simulink library "bcm"  (R2021b)
settings: Solver=VariableStepAuto  StartTime=0.0  StopTime=10.0  RelTol=1e-3
undefined symbols (not defined in the file or in its folder): ENUM_ANTITHEFT_ALARM, ENUM_ANTITHEFT_ARM, ENUM_ANTITHEFT_DISARM, ENUM_ANTITHEFT_WAIT, ENUM_GEARPOSNTOCAN_P, ENUM_PDKEYRAWLULOCK_INUNLOCK, ENUM_PDKEYRAWPS_INPS, ENUM_POWERSTA_ON, ENUM_POWERSTA_READY, ENUM_POWERSTA_STANDBY, ENUM_PWRSTASW_ON, ENUM_PWRSTASW_READY, ENUM_VEHICLETYPE_D21, ENUM_VEHICLETYPE_D31F25, ENUM_VEHICLETYPE_D31HAWD, ENUM_VEHICLETYPE_D31HRWD, ENUM_VEHICLETYPE_D31L24, FALSE, KBCM_ACCSwcPrsTmr_s, KBCM_ALMBrightnessDark_enum, KBCM_AmbBlue_enum, KBCM_AmbBreathT_ms, KBCM_AmbGreen_enum, KBCM_AmbMidPple_enum, KBCM_AmbRed_enum, KBCM_AmbTempCtrlEN_flg, KBCM_AmbTempT_s, KBCM_AmbWelModeENWait_s, KBCM_Antitheft_enum_ovrdflg, KBCM_Antitheft_enum_ovrdval, KBCM_APMDoorCtrlSta_flg_ovrdflg, KBCM_APMDoorCtrlSta_flg_ovrdval, KBCM_CmdKeepT_s, KBCM_CSWLightRstDebT_s, KBCM_CSWTurnLPRstT_s, KBCM_DelayTSW_flg, KBCM_DiagDRLOFF_flg, KBCM_DiagFLTC_mA, KBCM_DiagFMHT_s, KBCM_DiagFRTC_mA, KBCM_DiagRLTC_mA, KBCM_DiagRRTC_mA, KBCM_DrAPMRetryTimes_cnt, KBCM_DrOpenWdwOT_s, KBCM_DrOpenWdwReady_s, KBCM_ESSOffT_ms, KBCM_ESSOnT_ms, KBCM_FDCDKCReDetectT_K, KBCM_FDCDKCUSSFilterT_K, KBCM_HandleLampKeepT_s, KBCM_IVIRstHoldT_ms, KBCM_IVIRstTriggerT_ms, KBCM_ONDelayT_ms, KBCM_RAPSAbnFlashOFFT_ms, KBCM_RAPSAbnFlashONT_ms, KBCM_ReDetectT_K, KBCM_RightHandDriveEN_flg, KBCM_RLSLowSpdFilterT_s, KBCM_RmLampKeep_min, KBCM_RmLpKeyInT_s ... (+37)
libraries: simulink x389, $bdroot x11, hcu_lib x2
(part 13 of 13)

== stateflow chart bcm/BCM/BCM/Amb/AmbientLight ==
  state TempControl [parallel]
    settings: executionOrder=12
    state TempUP
      en:VBCM_AmbTemp_enum=1;
    state Wait
    state StandBy
      en:VBCM_AmbTemp_enum=0;
    state TempDN
      en:VBCM_AmbTemp_enum=2;
    (default) -> TempControl.StandBy
    TempControl -> TempUP [order 1] : [hasChanged(VBCM_TempUP_flg) && VBCM_TempUP_flg]
    TempUP -> TempControl.Wait : [!VBCM_TempUP_flg]
    TempControl.Wait -> TempControl.StandBy : [after(KBCM_AmbTempT_s,tick)]
    TempDN -> TempControl.Wait : [!VBCM_TempDN_flg]
    TempControl -> TempDN [order 2] : [hasChanged(VBCM_TempDN_flg) && VBCM_TempDN_flg]
  state OutputColor [parallel]
    settings: executionOrder=1
    (default) -> (junction 25)
    OutputColor -> (junction 25)
    (junction 25) -> (junction 947) [order 1] : [VINP_AmbLinkDriSta_flg]
    (junction 947) -> (junction 948) [order 1] : [VINP_IVISnowModeCmd_flg == 1]
        | {VBCM_AmbLightColor_enum = KBCM_AmbMidPurple_enum;}
    (junction 25) -> (junction 200) [order 2] : {VBCM_AmbLightColor_enum=VINP_AmbColorSta_enum;}
    (junction 947) -> (junction 28) [order 2]
    (junction 28) -> (junction 33) [order 1] : [VINP_IVIPWModeReq_enum==1]....
        | {VBCM_AmbLightColor_enum=KBCM_AmbRed_enum;}
    (junction 28) -> (junction 35) [order 2]
    (junction 35) -> (junction 37) [order 1] : [VINP_IVIPWModeReq_enum==2]....
        | {VBCM_AmbLightColor_enum=KBCM_AmbGreen_enum;}
    (junction 35) -> (junction 39) [order 2]
    (junction 39) -> (junction 41) : {VBCM_AmbLightColor_enum=KBCM_AmbBlue_enum;}
  state LampPower [parallel]
    settings: executionOrder=4
    state LampON
      state WaitForLampPwrON
        en:VBCM_LampPwr_flg=1;
      state LampPwrON
        en:VBCM_LampPwrReady_flg=true;
      (default) -> WaitForLampPwrON
      WaitForLampPwrON -> LampPwrON : after(5,tick)
    state OFF
      en:VBCM_LampPwr_flg=0;
      VBCM_LampPwrReady_flg=false;
    (default) -> LampPower.OFF
    LampPower.OFF -> LampON : [VBCM_WakeUp_flg==1||VPMM_PwrSta_enum>0]
    LampON -> LampPower.OFF : [VBCM_WakeUp_flg==0&&VPMM_PwrSta_enum==0]
  state WelcomeModeEnable [parallel]
    settings: executionOrder=13
    state WelcomeModeDisable
      en:
      VBCM_WelcomrModeEN_flg = FALSE;
    state WelcomrModeEnable
      state Wait
      state Enable
        en:
        VBCM_WelcomrModeEN_flg = TRUE;
      (default) -> WelcomeModeEnable.WelcomrModeEnable.Wait
      WelcomeModeEnable.WelcomrModeEnable.Wait -> Enable : [after(KBCM_AmbWelModeENWait_s, tick)]
    (default) -> WelcomeModeDisable
    WelcomeModeDisable -> WelcomeModeEnable.WelcomrModeEnable.Wait : [VPMM_PwrSta_enum > 3]
    WelcomrModeEnable -> WelcomeModeDisable : [VPMM_PwrSta_enum <= 3]
  state SOCDet [parallel]
    settings: executionOrder=5
    state ON
      state SOCOK
        en:SOCWarning=0;
      state SOCWarning1
      state SOCWarning2
        en:SOCWarning=1;
      (default) -> (junction 516)
      (junction 516) -> SOCOK [order 1] : [VINP_HVBattSOCDis_pct>5]
      (junction 516) -> (junction 518) [order 2]
      SOCOK -> SOCWarning1 : [VINP_HVBattSOCDis_pct<=5]....
          | {SOCWarning=1;}
      SOCWarning1 -> SOCOK [order 1] : [VINP_HVBattSOCDis_pct>5]
      (junction 518) -> SOCWarning1 [order 1] : [VINP_HVBattSOCDis_pct>=1]....
          | {SOCWarning=1;}
      (junction 518) -> (junction 521) [order 2]
      SOCWarning2 -> SOCWarning1 : [VINP_HVBattSOCDis_pct>=1]
      SOCWarning1 -> SOCWarning2 [order 2] : [VINP_HVBattSOCDis_pct<1]
      (junction 521) -> SOCWarning2
    state OFF
      en:SOCWarning=0;
    (default) -> SOCDet.OFF
    SOCDet.OFF -> SOCDet.ON : [VINP_AmbFunEN_flg&&....
        | VINP_AmbPwrWarnEN_flg]
    SOCDet.ON -> SOCDet.OFF : [!VINP_AmbPwrWarnEN_flg||....
        | !VINP_AmbFunEN_flg]
  state OutputBrightness [parallel]
    settings: executionOrder=3
    state ON
      (default) -> (junction 92)
      OutputBrightness.ON -> (junction 92) [order 1] : [VBCM_LampPwrReady_flg]
      (junction 92) -> (junction 90) [order 1] : [VINP_IVINightModeSta_flg&&VBCM_PosLamp_flg||VPMM_PwrSta_enum<=3]....
          | {VBCM_AmbLightBrightness_enum=KBCM_ALMBrightnessDark_enum;}
      (junction 92) -> (junction 203) [order 2]
      (junction 203) -> (junction 324) [order 1] : [!VINP_IVINightModeSta_flg&&VBCM_PosLamp_flg&&VINP_AmbDimEN_flg]....
          | {VBCM_AmbLightBrightness_enum=VINP_AmbBrightnessSta_enum/2;}
      (junction 203) -> (junction 208) [order 2] : {VBCM_AmbLightBrightness_enum=VINP_AmbBrightnessSta_enum;}
    state OFF
      en:VBCM_AmbLightBrightness_enum=0;
    (default) -> OutputBrightness.OFF
    OutputBrightness.OFF -> OutputBrightness.ON : [VINP_AmbFunEN_flg]
    OutputBrightness.ON -> OutputBrightness.OFF [order 1] : [!VINP_AmbFunEN_flg]
  state WelcomeMode [parallel]
    settings: executionOrder=2
    state Arm
      en:VBCM_Welcome_flg=0;
    state Disarm
      state WaitForDoorOpen
      state WaitForWelcomeModeEN
      state DoorOpen
        en:
        VBCM_Welcome_flg=1;
        on after(KBCM_AmbBreathT_tick,tick):
        VBCM_Welcome_flg=0;
      (default) -> (junction 498)
      (junction 498) -> WaitForDoorOpen [order 2]
      (junction 498) -> WaitForWelcomeModeEN [order 1] : [VINP_AllDoorSW_flg || ....
          | VPMM_PwrSta_enum>3]
      WaitForDoorOpen -> WaitForWelcomeModeEN : [VINP_AllDoorSW_flg || ....
          | VPMM_PwrSta_enum>3]
      WaitForWelcomeModeEN -> DoorOpen : [VBCM_WelcomrModeEN_flg]
    (default) -> (junction 492)
    (junction 492) -> Disarm [order 1] : [EEP_AntitheftSta==0]
    (junction 492) -> Arm [order 2]
    Arm -> Disarm : [AntitheftSta==0]
    Disarm -> Arm : [AntitheftSta!=0]
  state WarningLamp1 [parallel]
    settings: executionOrder=11
    state StandBy
    state Wait
    (default) -> (junction 549)
    WarningLamp1.StandBy -> (junction 549)
    (junction 549) -> (junction 504)
    (junction 545) -> WarningLamp1.StandBy
    (junction 504) -> (junction 545) [order 1] : [VINP_AmbFunEN_flg&&VBCM_Welcome_flg&&VINP_AmbWelEN_flg]{VBCM_AmblightBreath1_enum=1;}
    (junction 504) -> (junction 527) [order 2]
    (junction 543) -> (junction 545)
    WarningLamp1.Wait -> (junction 543) : [after(KBCM_AmbBreathT_tick,tick)]
    (junction 527) -> WarningLamp1.Wait [order 1] : [VINP_AmbFunEN_flg&&SOCWarning==1]....
        | {SOCWarning=0;VBCM_AmblightBreath1_enum=2;}
    (junction 527) -> (junction 900) [order 2]
    (junction 903) -> (junction 543)
    (junction 900) -> (junction 903) [order 1] : [VINP_VehicleType_enum != ENUM_VEHICLETYPE_D31L24 && ...
        | VINP_AmbFunEN_flg && KBCM_AmbTempCtrlEN_flg && VBCM_AmbTemp_enum==1]
        | {VBCM_AmblightBreath1_enum =4 ;}
    (junction 900) -> (junction 901) [order 2]
    (junction 902) -> (junction 903)
    (junction 901) -> (junction 902) [order 1] : [VINP_VehicleType_enum != ENUM_VEHICLETYPE_D31L24 && ...
        | VINP_AmbFunEN_flg && KBCM_AmbTempCtrlEN_flg && VBCM_AmbTemp_enum==2]
        | {VBCM_AmblightBreath1_enum =5 ;}
    (junction 901) -> (junction 537) [order 2]
    (junction 542) -> (junction 902)
    (junction 537) -> (junction 542) : {SOCWarning=0;VBCM_AmblightBreath1_enum=0;}
  state WarningLamp3 [parallel]
    settings: executionOrder=7
    state StandBy
    state Wait
    (default) -> (junction 576)
    WarningLamp3.StandBy -> (junction 576)
    (junction 576) -> (junction 577)
    (junction 578) -> WarningLamp3.StandBy
    (junction 577) -> (junction 578) [order 1] : [VINP_AmbFunEN_flg&&VBCM_Welcome_flg&&VINP_AmbWelEN_flg]{VBCM_AmblightBreath3_enum=1;}
    (junction 577) -> (junction 597) [order 2]
    (junction 598) -> (junction 578)
    (junction 597) -> (junction 598) [order 1] : [VINP_AmbFunEN_flg&&VINP_AmbODAEN_flg&&....
        | ((VINP_SRRODASoundL_flg==1&&VBCM_FLDoorSW_flg==1)||VINP_SRRBSDWarnL_enum==2)]
        | {VBCM_AmblightBreath3_enum=3;}
    (junction 597) -> (junction 579) [order 2]
    (junction 580) -> (junction 598)
    (junction 579) -> WarningLamp3.Wait [order 1] : [VINP_AmbFunEN_flg&&SOCWarning==1]....
        | {VBCM_AmblightBreath3_enum=2;}
    WarningLamp3.Wait -> (junction 580) : [after(KBCM_AmbBreathT_tick,tick)]
    (junction 579) -> (junction 581) [order 2]
    (junction 582) -> (junction 580)
    (junction 581) -> (junction 582) : {VBCM_AmblightBreath3_enum=0;}
  state WarningLamp5 [parallel]
    settings: executionOrder=9
    state StandBy
    state Wait
    (default) -> (junction 630)
    WarningLamp5.StandBy -> (junction 630)
    (junction 630) -> (junction 631)
    (junction 632) -> WarningLamp5.StandBy
    (junction 631) -> (junction 632) [order 1] : [VINP_AmbFunEN_flg&&VBCM_Welcome_flg&&VINP_AmbWelEN_flg]{VBCM_AmblightBreath5_enum=1;}
    (junction 631) -> (junction 633) [order 2]
    (junction 634) -> (junction 632)
    (junction 633) -> (junction 634) [order 1] : [VINP_AmbFunEN_flg&&VINP_AmbODAEN_flg&&VINP_SRRODASoundL_flg==1&&VINP_RLDoorSW_flg==1]....
        | {VBCM_AmblightBreath5_enum=3;}
    (junction 633) -> (junction 635) [order 2]
    (junction 636) -> (junction 634)
    (junction 635) -> WarningLamp5.Wait [order 1] : [VINP_AmbFunEN_flg&&SOCWarning==1]....
        | {VBCM_AmblightBreath5_enum=2;}
    WarningLamp5.Wait -> (junction 636) : [after(KBCM_AmbBreathT_tick,tick)]
    (junction 635) -> (junction 637) [order 2]
    (junction 638) -> (junction 636)
    (junction 637) -> (junction 638) : {VBCM_AmblightBreath5_enum=0;}
  state WarningLamp2 [parallel]
    settings: executionOrder=6
    state StandBy
    state Wait
    (default) -> (junction 554)
    WarningLamp2.StandBy -> (junction 554)
    (junction 554) -> (junction 555)
    (junction 556) -> WarningLamp2.StandBy
    (junction 555) -> (junction 556) [order 1] : [VINP_AmbFunEN_flg&&VBCM_Welcome_flg&&VINP_AmbWelEN_flg]{VBCM_AmblightBreath2_enum=1;}
    (junction 555) -> (junction 557) [order 2]
    (junction 558) -> (junction 556)
    (junction 557) -> WarningLamp2.Wait [order 1] : [VINP_AmbFunEN_flg&&SOCWarning==1]....
        | {VBCM_AmblightBreath2_enum=2;}
    WarningLamp2.Wait -> (junction 558) : [after(KBCM_AmbBreathT_tick,tick)]
    (junction 557) -> (junction 910) [order 2]
    (junction 912) -> (junction 558)
    (junction 910) -> (junction 912) [order 1] : [VINP_VehicleType_enum != ENUM_VEHICLETYPE_D31L24 && ...
        | VINP_AmbFunEN_flg && KBCM_AmbTempCtrlEN_flg && VBCM_AmbTemp_enum==1]
        | {VBCM_AmblightBreath2_enum =4 ;}
    (junction 910) -> (junction 911) [order 2]
    (junction 913) -> (junction 912)
    (junction 911) -> (junction 913) [order 1] : [VINP_VehicleType_enum != ENUM_VEHICLETYPE_D31L24 && ...
        | VINP_AmbFunEN_flg && KBCM_AmbTempCtrlEN_flg && VBCM_AmbTemp_enum==2]
        | {VBCM_AmblightBreath2_enum =5 ;}
    (junction 911) -> (junction 559) [order 2]
    (junction 560) -> (junction 913)
    (junction 559) -> (junction 560) : {VBCM_AmblightBreath2_enum=0;}
  state WarningLamp4 [parallel]
    settings: executionOrder=8
    state StandBy
    state Wait
    (default) -> (junction 603)
    WarningLamp4.StandBy -> (junction 603)
    (junction 603) -> (junction 604)
    (junction 605) -> WarningLamp4.StandBy
    (junction 604) -> (junction 605) [order 1] : [VINP_AmbFunEN_flg&&VBCM_Welcome_flg&&VINP_AmbWelEN_flg]{VBCM_AmblightBreath4_enum=1;}
    (junction 604) -> (junction 606) [order 2]
    (junction 607) -> (junction 605)
    (junction 606) -> (junction 607) [order 1] : [VINP_AmbFunEN_flg&&VINP_AmbODAEN_flg&&....
        | ((VINP_SRRODASoundR_flg==1&&VBCM_FRDoorSW_flg==1)||VINP_SRRBSDWarnR_enum==2)]
        | {VBCM_AmblightBreath4_enum=3;}
    (junction 606) -> (junction 608) [order 2]
    (junction 609) -> (junction 607)
    (junction 608) -> WarningLamp4.Wait [order 1] : [VINP_AmbFunEN_flg&&SOCWarning==1]....
        | {VBCM_AmblightBreath4_enum=2;}
    WarningLamp4.Wait -> (junction 609) : [after(KBCM_AmbBreathT_tick,tick)]
    (junction 608) -> (junction 610) [order 2]
    (junction 611) -> (junction 609)
    (junction 610) -> (junction 611) : {VBCM_AmblightBreath4_enum=0;}
  state WarningLamp6 [parallel]
    settings: executionOrder=10
    state StandBy
    state Wait
    (default) -> (junction 657)
    WarningLamp6.StandBy -> (junction 657)
    (junction 657) -> (junction 658)
    (junction 659) -> WarningLamp6.StandBy
    (junction 658) -> (junction 659) [order 1] : [VINP_AmbFunEN_flg&&VBCM_Welcome_flg&&VINP_AmbWelEN_flg]{VBCM_AmblightBreath6_enum=1;}
    (junction 658) -> (junction 660) [order 2]
    (junction 661) -> (junction 659)
    (junction 660) -> (junction 661) [order 1] : [VINP_AmbFunEN_flg&&VINP_AmbODAEN_flg&&VINP_SRRODASoundR_flg==1&&VINP_RRDoorSW_flg==1]....
        | {VBCM_AmblightBreath6_enum=3;}
    (junction 660) -> (junction 662) [order 2]
    (junction 663) -> (junction 661)
    (junction 662) -> WarningLamp6.Wait [order 1] : [VINP_AmbFunEN_flg&&SOCWarning==1]....
        | {VBCM_AmblightBreath6_enum=2;}
    WarningLamp6.Wait -> (junction 663) : [after(KBCM_AmbBreathT_tick,tick)]
    (junction 662) -> (junction 664) [order 2]
    (junction 665) -> (junction 663)
    (junction 664) -> (junction 665) : {VBCM_AmblightBreath6_enum=0;}
  data: VINP_AmbWelEN_flg input boolean; VINP_AmbColorSta_enum input uint8; VINP_AmbDimEN_flg input boolean; VINP_AmbFunEN_flg input boolean; KBCM_ALMBrightnessDark_enum input; VINP_AmbODAEN_flg input boolean; KBCM_AmbGreen_enum input; VINP_AmbPwrWarnEN_flg input boolean; KBCM_AmbRed_enum input; VINP_AmbBrightnessSta_enum input uint8; VINP_AmbLinkDriSta_flg input boolean; VINP_IVIPWModeReq_enum input uint8; KBCM_AmbBlue_enum input; KBCM_AmbBreathT_tick input; VINP_IVINightModeSta_flg input boolean; VBCM_PosLamp_flg input boolean; VINP_AllDoorSW_flg input boolean; VPMM_PwrSta_enum input uint8; VBCM_LampPwr_flg output boolean; VBCM_WakeUp_flg input boolean; VBCM_AmbLightBrightness_enum output uint8 =0; VBCM_AmbLightColor_enum output uint8 =0; SOCWarning local boolean; AntitheftSta input uint8; EEP_AntitheftSta input uint8; VBCM_FLDoorSW_flg input; VBCM_FRDoorSW_flg input; VINP_RLDoorSW_flg input; VINP_RRDoorSW_flg input; VINP_HVBattSOCDis_pct input uint8; VINP_SRRBSDWarnL_enum input uint8; VINP_SRRBSDWarnR_enum input uint8; VINP_SRRODASoundL_flg input boolean; VINP_VehicleType_enum input; VINP_SRRODASoundR_flg input boolean; VBCM_AmblightBreath1_enum output uint8; VBCM_AmblightBreath2_enum output uint8; VBCM_AmblightBreath3_enum output uint8; VBCM_AmblightBreath4_enum output uint8; VBCM_AmblightBreath5_enum output uint8; VBCM_AmblightBreath6_enum output uint8; VBCM_Welcome_flg local boolean; VBCM_TempDN_flg input; VBCM_TempUP_flg input; VINP_IVISnowModeCmd_flg input; KBCM_AmbTempCtrlEN_flg input; VBCM_AmbTemp_enum local uint8; KBCM_AmbTempT_s input; VBCM_LampPwrReady_flg output boolean =0; ENUM_VEHICLETYPE_D31L24 parameter; VBCM_WelcomrModeEN_flg local boolean; FALSE parameter; TRUE parameter; KBCM_AmbWelModeENWait_s input; KBCM_AmbMidPurple_enum input

== stateflow chart bcm/BCM/BCM/BCM_WAKE_MODULE/Chart ==
  state SleepReqJudge
    (default) -> (junction 3) : {
        |  VBCM_SleepReqLAST_flg = TRUE;
        |  VBCM_ConditionTimer_s = 0;
        |  }
    SleepReqJudge -> (junction 3)
    (junction 3) -> (junction 11) [order 2]
    (junction 3) -> (junction 7) [order 1] : [VBCM_SlpConditionMeet_flg]
    (junction 11) -> (junction 31) : {
        |   VBCM_SleepReq_flg = FALSE;
        |   VBCM_SleepReqLAST_flg = VBCM_SleepReq_flg;
        |   VBCM_ConditionTimer_s = 0;
        | }
    (junction 7) -> (junction 17) [order 2]
    (junction 7) -> (junction 26) [order 1] : [VBCM_SleepReqLAST_flg]
    (junction 17) -> (junction 19) : {VBCM_ConditionTimer_s += task_time_s;}
    (junction 19) -> (junction 31) [order 2]
    (junction 19) -> (junction 24) [order 1] : [VBCM_ConditionTimer_s >= KBCM_SlpDebounceTime_s]
    (junction 31) -> (junction 13)
    (junction 24) -> (junction 26)
    (junction 26) -> (junction 29) : {
        |  VBCM_SleepReq_flg = TRUE;
        |  VBCM_SleepReqLAST_flg = VBCM_SleepReq_flg;
        |  VBCM_ConditionTimer_s = 0;
        | }
    (junction 29) -> (junction 13)
  (default) -> SleepReqJudge
  data: TRUE parameter; VBCM_SleepReq_flg output boolean; VBCM_ConditionTimer_s local single; VBCM_SlpConditionMeet_flg input; FALSE parameter; VBCM_SleepReqLAST_flg local boolean; task_time_s input; KBCM_SlpDebounceTime_s input

== stateflow chart bcm/BCM/BCM/IVI Reset/Chart ==
  state sRelease
    en:
    VBCM_IVIRST_flg = FALSE;
  state sPress
  state sIVI_RESET_SEND
    en:
    VBCM_IVIRST_flg = TRUE;
  state sSTOP
    en:
    VBCM_IVIRST_flg = FALSE;
  (default) -> sRelease
  sRelease -> sPress : [VINP_SWCmodeSta_flg]
  sPress -> sRelease [order 1] : [!VINP_SWCmodeSta_flg]
  sPress -> sIVI_RESET_SEND [order 2] : [after(KBCM_IVIRstTriggerT_ms,tick)]
  sIVI_RESET_SEND -> sSTOP : [after(KBCM_IVIRstHoldT_ms,tick)]
  sSTOP -> sRelease : [!VINP_SWCmodeSta_flg]
  data: KBCM_IVIRstHoldT_ms input; KBCM_IVIRstTriggerT_ms input; VINP_SWCmodeSta_flg input; VBCM_IVIRST_flg output; FALSE parameter; TRUE parameter

== stateflow chart bcm/BCM/BCM/PTG/Chart ==
  state Alarm
    en:
    VBCM_SPTGDet_flg=1;
  state NoDetected
    en:
    VBCM_SPTGDet_flg=0;
    VBCM_APSOpenPTG_flg=0;
  state WaitForDKC
  state DoorOpen
    en:
    VBCM_SPTGDet_flg=0;
    VBCM_APSOpenPTG_flg=1;
  state WaitforLeave
    en:
    VBCM_APSOpenPTG_flg=0;
    VBCM_SPTGDet_flg=0;
    state OutRange
    state InRange
    (default) -> InRange
    InRange -> OutRange : [(PASDRMR>=100 || PASDRML>=100) && (!TailgateSW)]
    OutRange -> InRange [order 1] : [(PASDRMR<100 && PASDRML<100) || TailgateSW]
  (junction 109) -> NoDetected [order 1] : [KBCM_DelayTSW_flg==0]{VBCM_u8DetectWaitT_s=0;}
  Alarm -> (junction 109) [order 1] : [hasChangedTo(KeyDetectedOut,0)....
      | &&....
      | KBCM_SPTGLeave_flg==1]
  (junction 109) -> (junction 70) [order 2]
  (junction 70) -> NoDetected : {VBCM_u8DetectWaitT_s=KBCM_SPTGDetectWaitT_s;}
  (junction 128) -> Alarm
  WaitForDKC -> (junction 128) [order 1] : [PDKeyAreaPTG==1]
  NoDetected -> NoDetected [order 2] : [VBCM_u8DetectWaitT_s>0]{VBCM_u8DetectWaitT_s=VBCM_u8DetectWaitT_s-1;}
  Alarm -> WaitforLeave [order 2] : [ShiftGearPosn!=0||....
      | VehSpeed>0||....
      | PwrSta==5||....
      | TailgateSW!=0||....
      | IVI_PTG_USSta_SW!=0||....
      | PDKeyAreaPTG!=1]
  Alarm -> WaitforLeave [order 3] : [DKCKeyPress]
  Alarm -> DoorOpen [order 4] : [after(KBCM_SPTGDetectT_sec*100,tick)]
  NoDetected -> WaitForDKC [order 1] : [hasChangedTo(KeyDetected,1)&&VBCM_u8DetectWaitT_s==0....
      | &&....
      | (ShiftGearPosn==0&&....
      | VehSpeed<=0&&....
      | PwrSta!=5&&....
      | TailgateSW==0&&....
      | IVI_PTG_USSta_SW==0)]
  DoorOpen -> WaitforLeave : [after(40,tick)]
  (default) -> WaitforLeave
  (junction 136) -> NoDetected [order 1] : [KBCM_DelayTSW_flg==0]{VBCM_u8DetectWaitT_s=0;}
  WaitForDKC -> (junction 136) [order 2] : [hasChangedTo(KeyDetectedOut,0)....
      | &&....
      | KBCM_SPTGLeave_flg==1]
  (junction 136) -> (junction 138) [order 2]
  WaitForDKC -> WaitforLeave [order 3] : [after(KBCM_SPTGWaitDKC_sec*100,tick)]
  (junction 138) -> NoDetected : {VBCM_u8DetectWaitT_s=100;}
  OutRange -> NoDetected [order 2] : after(KBCM_ReDetectT_K,tick)
  data: KBCM_DelayTSW_flg input; KeyDetected input; PASDRMR input; PASDRML input; PDKeyAreaPTG input; PwrSta input; KeyDetectedOut input; TailgateSW input; VehSpeed input; DKCKeyPress input; ShiftGearPosn input; IVI_PTG_USSta_SW input; VBCM_APSOpenPTG_flg output; VBCM_SPTGDet_flg output; VBCM_u8DetectWaitT_s local uint8 =0; KBCM_ReDetectT_K input =1; KBCM_SPTGDetectT_sec input; KBCM_SPTGLeave_flg input; KBCM_SPTGWaitDKC_sec input; KBCM_SPTGDetectWaitT_s input

== stateflow chart bcm/BCM/BCM/APM_Door/DoorAPM/window ==
  state Normal
    state DoorClose
      state NoResponse
      state PwrOpenReq
        en:CtrlCmd = 126;
      state WinClose
        en:CtrlCmd = 0;
        ex:CtrlCmd = 127;
      state StandBy
      (default) -> (junction 123)
      (junction 123) -> (junction 124) [order 1] : [ Val_Wdw_Opened > 8....
          | ||....
          | Val_Wdw_Opened <= 0 ]
      (junction 123) -> (junction 58) [order 2]
      (junction 124) -> Normal.DoorClose.NoResponse
      (junction 58) -> (junction 56) [order 1] : [!CANMsgValidGWZoneDR1....
          | ||....
          | !CANMsgValidGWZoneFR1]
      (junction 56) -> Normal.DoorClose.NoResponse [order 2]
      (junction 58) -> WinClose [order 2]
      (junction 56) -> Normal.DoorClose.PwrOpenReq [order 1] : [DrAPMRetryCnt<KBCM_DrAPMRetryTimes_cnt]
      (junction 130) -> Normal.DoorClose.NoResponse
      Normal.DoorClose.PwrOpenReq -> WinClose [order 1] : [CANMsgValidGWZoneDR1....
          | &&....
          | CANMsgValidGWZoneFR1]
      WinClose -> Normal.DoorClose.StandBy : [Val_Wdw_Opened <= 0 || ...
          | after(DrOpenWdwOT_K,tick)]
      Normal.DoorClose.PwrOpenReq -> (junction 99) [order 2]
      (junction 99) -> Normal.DoorClose.StandBy : [after(WaitAPMPwr_K,tick)]
          | {CtrlCmd=127;
          | DrAPMRetryCnt=DrAPMRetryCnt+1;}
      Normal.DoorClose.StandBy -> (junction 130) [order 1] : [hasChanged(Val_Wdw_Opened)]
    state DoorOpen
      state NoResponse
      state WinOpen
        en:CtrlCmd = 6;
        ex:CtrlCmd = 127;
      state PwrOpenReq
        en:CtrlCmd = 126;
      state StandBy
      (default) -> (junction 48)
      (junction 48) -> (junction 120) [order 1]
      (junction 48) -> (junction 51) [order 2] : [!CANMsgValidGWZoneDR1....
          | ||....
          | !CANMsgValidGWZoneFR1]
      (junction 51) -> Normal.DoorOpen.NoResponse [order 2]
      (junction 120) -> Normal.DoorOpen.StandBy : [ Val_Wdw_Opened > 0 ]
      (junction 48) -> WinOpen [order 3]
      (junction 51) -> Normal.DoorOpen.PwrOpenReq [order 1] : [DrAPMRetryCnt<KBCM_DrAPMRetryTimes_cnt]
      Normal.DoorOpen.PwrOpenReq -> WinOpen [order 1] : [CANMsgValidGWZoneDR1....
          | &&....
          | CANMsgValidGWZoneFR1]
      Normal.DoorOpen.PwrOpenReq -> (junction 102) [order 2]
      WinOpen -> Normal.DoorOpen.StandBy : [Val_Wdw_Opened >= 6 || ...
          | after(DrOpenWdwOT_K,tick)]
      (junction 102) -> Normal.DoorOpen.StandBy : [after(WaitAPMPwr_K,tick)]
          | {CtrlCmd=127;
          | DrAPMRetryCnt=DrAPMRetryCnt+1;}
    state Reverse
    (default) -> DoorClose
    (junction 8) -> DoorClose [order 1] : [!DoorSW]
    (junction 8) -> DoorOpen [order 2]
    Reverse -> (junction 8) : [CtrlCmd_Ready]
    (junction 21) -> Reverse [order 2]
    DoorClose -> (junction 21) : [DoorSW]
        | {DrAPMRetryCnt=0;}
    (junction 21) -> DoorOpen [order 1] : [CtrlCmd_Ready]
    (junction 29) -> (junction 21) [order 2]
    (junction 29) -> DoorClose [order 1] : [CtrlCmd_Ready]
    DoorOpen -> (junction 29) : [!DoorSW]
        | {DrAPMRetryCnt=0;}
    (junction 94) -> (junction 29)
    Normal.DoorClose.StandBy -> (junction 94) [order 2] : [ Val_Wdw_Opened <= 8 && Val_Wdw_Opened > 0 ]
    Normal.DoorOpen.StandBy -> (junction 94) [order 2] : [ Val_Wdw_Opened <= 0 ]
  state ManualOpen
    en:
    CtrlCmd = 127;
  state IVICmdSend
    en:
    CtrlCmd = ControlCommand_Buf;
  state CommandRst
    en:
    CtrlCmd=127;
  (default) -> ManualOpen
  ManualOpen -> (junction 65) [order 2]
  Normal -> (junction 65) [order 1]
  (junction 65) -> (junction 66) : [hasChangedFrom(ControlCommand, 127)]
      | {ControlCommand_Buf = ControlCommand;}
  (junction 66) -> (junction 79) [order 2]
  (junction 79) -> IVICmdSend
  (junction 66) -> CommandRst [order 1] : [!CtrlCmd_Ready]
  CommandRst -> IVICmdSend : [CtrlCmd_Ready]
  IVICmdSend -> ManualOpen : [after(12,tick)]
  Normal -> ManualOpen [order 2] : [!APMDoorControlSta]
  ManualOpen -> Normal.DoorClose.StandBy [order 1] : [APMDoorControlSta]
      | {DrAPMRetryCnt=0;}
  Normal.DoorOpen.StandBy -> ManualOpen [order 1] : [( hasChanged(Val_Wdw_Opened) && ( Val_Wdw_Opened>=8 ) ) && after(KBCM_WdwManualDetT_K,tick)]
  data: DoorSW input boolean; Val_Wdw_Opened input uint8; WaitAPMPwr_K input uint8; APMDoorControlSta input; CtrlCmd_Ready input; ControlCommand input; DrOpenWdwOT_K input uint8; CtrlCmd output uint8; ControlCommand_Buf local uint8; KBCM_WdwManualDetT_K input; CANMsgValidGWZoneDR1 input boolean; CANMsgValidGWZoneFR1 input boolean; KBCM_DrAPMRetryTimes_cnt input; DrAPMRetryCnt local uint8 =0

== stateflow chart bcm/BCM/BCM/Personal_Setting/ACC/Chart ==
  state ACC_Disable
    en:
    VBCM_LRightStaCmd_flg = VINP_SWC2LRightSta_flg;
    VBCM_LLeftStaCmd_flg = VINP_SWC2LLeftSta_flg;
    VBCM_ACCSetUpCnt_cnt = 0;
    VBCM_ACCSetDnCnt_cnt = 0;
    du:
    VBCM_LRightStaCmd_flg = VINP_SWC2LRightSta_flg;
    VBCM_LLeftStaCmd_flg = VINP_SWC2LLeftSta_flg;
  state ACC_Sync
    en:
    VBCM_LRightStaCmd_flg = 0;
    VBCM_LLeftStaCmd_flg = 0;
  state UP_Press
    en:
    VBCM_LRightStaCmd_flg = 1;
    VBCM_LLeftStaCmd_flg = 0;
  state DN_Press
    en:
    en:
    VBCM_LRightStaCmd_flg = 0;
    VBCM_LLeftStaCmd_flg = 1;
  state ACC_Enable
    en:
    VBCM_LRightStaCmd_flg = 0;
    VBCM_LLeftStaCmd_flg = 0;
    du:
    VBCM_LRightStaCmd_flg = 0;
    VBCM_LLeftStaCmd_flg = 0;
  (default) -> ACC_Disable
  ACC_Sync -> ACC_Disable [order 1] : [!VBCM_ACCChangeEnable_flg]
  ACC_Sync -> UP_Press [order 2] : [after(KBCM_ACCSwcPrsTmr_s,tick)....
      | &&....
      | VBCM_ACCSetUpCnt_cnt > 0]
      | {VBCM_ACCSetUpCnt_cnt = VBCM_ACCSetUpCnt_cnt -1;}
  UP_Press -> ACC_Sync : [after(KBCM_ACCSwcPrsTmr_s,tick)]
  DN_Press -> ACC_Sync : [after(KBCM_ACCSwcPrsTmr_s,tick)]
  ACC_Sync -> DN_Press [order 3] : [after(KBCM_ACCSwcPrsTmr_s,tick)&&....
      | VBCM_ACCSetDnCnt_cnt > 0]
      | {VBCM_ACCSetDnCnt_cnt = VBCM_ACCSetDnCnt_cnt -1;}
  ACC_Sync -> ACC_Enable [order 4] : [VBCM_ACCSetUpCnt_cnt == 0....
      | &&....
      | VBCM_ACCSetDnCnt_cnt == 0....
      | &&....
      | after(KBCM_WaitACCChange_s,tick)]
  ACC_Enable -> ACC_Sync [order 2] : [VINP_TimeGapLevel_enum <= 4 && VINP_TimeGapLevel_enum > VBCM_TimeGapLevelSta_enum]
      | {VBCM_ACCSetUpCnt_cnt = 0;
      |  VBCM_ACCSetDnCnt_cnt = VINP_TimeGapLevel_enum - VBCM_TimeGapLevelSta_enum;}
  ACC_Enable -> ACC_Sync [order 3] : [VINP_TimeGapLevel_enum <= 4 && VINP_TimeGapLevel_enum < VBCM_TimeGapLevelSta_enum]
      | {VBCM_ACCSetUpCnt_cnt = VBCM_TimeGapLevelSta_enum - VINP_TimeGapLevel_enum;....
      |  VBCM_ACCSetDnCnt_cnt = 0;}
  ACC_Disable -> ACC_Enable : [VBCM_ACCChangeEnable_flg]
  ACC_Enable -> ACC_Disable [order 1] : [!VBCM_ACCChangeEnable_flg]
  data: VBCM_ACCChangeEnable_flg input; VBCM_LRightStaCmd_flg output boolean; VBCM_LLeftStaCmd_flg output boolean; VINP_TimeGapLevel_enum input; VBCM_TimeGapLevelSta_enum input; VINP_SWC2LRightSta_flg input; VINP_SWC2LLeftSta_flg input; VBCM_ACCSetDnCnt_cnt local uint8; VBCM_ACCSetUpCnt_cnt local uint8; KBCM_ACCSwcPrsTmr_s input; KBCM_WaitACCChange_s input

== stateflow chart bcm/BCM/BCM/CSW/Chart ==
  state OFF
    en:CSW2TSw=0;
  state LeftControl
    en:CSW2TSw=1;
    state LightLeft
      state Debounce
      state Hold
      state StandBy
      (default) -> LeftControl.LightLeft.StandBy
      LeftControl.LightLeft.StandBy -> LeftControl.LightLeft.Debounce [order 1] : [hasChanged(VINP_CSW2TurnSwSta_enum) &&....
          | VINP_CSW2TurnSwSta_enum == 3]
      LeftControl.LightLeft.StandBy -> LeftControl.LightLeft.Hold [order 2] : [after(tset,tick) ||....
          | hasChanged(VINP_CSW2TurnSwSta_enum) &&....
          | VINP_CSW2TurnSwSta_enum == 1]
    state Left
      state Debounce
      state StandBy
      (default) -> LeftControl.Left.StandBy
      LeftControl.Left.StandBy -> LeftControl.Left.Debounce [order 1] : [hasChanged(VINP_CSW2TurnSwSta_enum) &&....
          | VINP_CSW2TurnSwSta_enum == 3]
      LeftControl.Left.StandBy -> (junction 119) [order 2] : [hasChanged(VINP_CSW2TurnSwSta_enum) &&....
          | VINP_CSW2TurnSwSta_enum == 1]
    (default) -> LightLeft
    (junction 119) -> LeftControl.LightLeft.Hold
    LightLeft -> Left : [VINP_CSW2TurnSwSta_enum == 2]
  state RESET
    en:CSW2TSw = 0;
  state RightControl
    en:CSW2TSw=2;
    state Right
      state Debounce
      state StandBy
      (default) -> RightControl.Right.StandBy
      RightControl.Right.StandBy -> RightControl.Right.Debounce [order 1] : [hasChanged(VINP_CSW2TurnSwSta_enum) &&....
          | VINP_CSW2TurnSwSta_enum == 1]
      RightControl.Right.StandBy -> (junction 153) [order 2] : [hasChanged(VINP_CSW2TurnSwSta_enum) &&....
          | VINP_CSW2TurnSwSta_enum == 3]
    state LightRight
      state Hold
      state Debounce
      state StandBy
      (default) -> RightControl.LightRight.StandBy
      RightControl.LightRight.StandBy -> RightControl.LightRight.Debounce [order 1] : [hasChanged(VINP_CSW2TurnSwSta_enum) &&....
          | VINP_CSW2TurnSwSta_enum == 1]
      RightControl.LightRight.StandBy -> RightControl.LightRight.Hold [order 2] : [after(tset,tick) ||....
          | hasChanged(VINP_CSW2TurnSwSta_enum) &&....
          | VINP_CSW2TurnSwSta_enum == 3]
    (junction 153) -> RightControl.LightRight.Hold
    LightRight -> Right : [VINP_CSW2TurnSwSta_enum == 4 ]
    (default) -> LightRight
  (default) -> OFF
  LeftControl.LightLeft.Debounce -> OFF [order 1] : [VINP_CSW2TurnSwSta_enum != 3 && VINP_CSW2TurnSwSta_enum != 4]
  OFF -> (junction 110) [order 1] : [VINP_CSW2TurnSwSta_enum == 1]
  (junction 110) -> LeftControl [order 1] : [hasChanged(VINP_CSW2TurnSwSta_enum)]
  (junction 110) -> (junction 113) [order 2]
  (junction 113) -> LeftControl.LightLeft.Hold
  LeftControl.LightLeft.Debounce -> RESET [order 2] : [after(KBCM_CSWLightRstDebT_s,tick)]
  LeftControl.LightLeft.Hold -> OFF : [VINP_CSW2TurnSwSta_enum != 1]
  OFF -> Left [order 2] : [VINP_CSW2TurnSwSta_enum == 2]
  Left -> OFF : [LeftRelflg && VINP_CSW2TurnSwSta_enum != 1 && VINP_CSW2TurnSwSta_enum != 2]
  LeftControl.Left.Debounce -> OFF [order 1] : [VINP_CSW2TurnSwSta_enum != 3 && VINP_CSW2TurnSwSta_enum != 4]
  LeftControl.Left.Debounce -> RESET [order 2] : [after(KBCM_CSWLightRstDebT_s,tick)]
  RightControl -> LeftControl : [VINP_CSW2TurnSwSta_enum == 2]
  LeftControl -> RightControl : [VINP_CSW2TurnSwSta_enum == 4]
  RESET -> OFF : [ (VINP_CSW2TurnSwSta_enum != 1 && VINP_CSW2TurnSwSta_enum != 3) || after(KBCM_CSWTurnLPRstT_s,tick)]
  RightControl.Right.Debounce -> RESET [order 1] : [after(KBCM_CSWLightRstDebT_s,tick)]
  RightControl.LightRight.Debounce -> RESET [order 1] : [after(KBCM_CSWLightRstDebT_s,tick)]
  RightControl.Right.Debounce -> OFF [order 2] : [VINP_CSW2TurnSwSta_enum != 1 && VINP_CSW2TurnSwSta_enum != 2]
  OFF -> Right [order 4] : [ VINP_CSW2TurnSwSta_enum == 4 ]
  Right -> OFF : [ RightRelflg && VINP_CSW2TurnSwSta_enum != 3 && VINP_CSW2TurnSwSta_enum != 4 ]
  OFF -> (junction 183) [order 3] : [VINP_CSW2TurnSwSta_enum == 3]
  (junction 183) -> RightControl [order 1] : [hasChanged(VINP_CSW2TurnSwSta_enum)]
  (junction 183) -> (junction 179) [order 2]
  (junction 179) -> RightControl.LightRight.Hold
  RightControl.LightRight.Hold -> OFF : [ VINP_CSW2TurnSwSta_enum != 3 ]
  RightControl.LightRight.Debounce -> OFF [order 2] : [ VINP_CSW2TurnSwSta_enum != 1 && VINP_CSW2TurnSwSta_enum != 2 ]
  data: VINP_CSW2TurnSwSta_enum input uint8; LeftRelflg input boolean; RightRelflg input boolean; CSW2TSw output uint8; tset input uint16; KBCM_CSWLightRstDebT_s input; KBCM_CSWTurnLPRstT_s input
